simulink model "Encoder_B02"  (R2024b)
settings: Solver=FixedStepAuto  StartTime=0.0  StopTime=inf  FixedStep=0.01  RelTol=1e-3  EnableMultiTasking=on
libraries: stm32f4xxblockslib x10, stm32g4xxblockslib x9
settings Model: STM32="{\"EncoderBlockForG4\":[{\"ID\":\"Hi:51\"},{\"ID\":\"Hi:52\"},{\"ID\":\"Hi:61\"},{\"ID\":\"Hi:103\"},{\"ID\":\"Hi:104\"},{\"ID\":\"Hi:105\"},{\"ID\":\"Hi:147\"},{\"ID\":\"Hi:148\"},{\"ID\":\"Hi:149\"}],\"DigitalPortRead\":[{\"ID\":\"Hi:68\"},{\"ID\":\"Hi:69\"},{\"ID\":\"Hi:95\"},{\"ID\":\"Hi:96\"},{\"ID\":\"Hi:118\"},{\"ID\":\"Hi:119\"},{\"ID\":\"Hi:131\"},{\"ID\":\"Hi:132\"},{\"ID\":\"Hi:133\"},{\"ID\":\"Hi:134\"}]}"  SimulationMode=external  Creator=User  LastModifiedBy=User
settings OptimizationCC: DefaultParameterBehavior=Inlined  EnhancedBackFolding=on  PassReuseOutputArgsAs=Individual arguments  ZeroExternalMemoryAtStartup=off  ZeroInternalMemoryAtStartup=off  MaxStackSize=512  OptimizeBlockOrder=speed  DifferentSizesBufferReuse=on  OptimizationCustomize=off  EfficientTunableParamExpr=on
settings DebuggingCC: ParameterTunabilityLossMsg=error
settings HardwareCC: ProdBitPerPointer=32  ProdBitPerSizeT=32  ProdBitPerPtrDiffT=32  ProdLargestAtomicInteger=Long  ProdLargestAtomicFloat=Double  ProdWordSize=32  ProdLongLongMode=on  ProdHWDeviceType=ARM Compatible->ARM Cortex-M
settings SFSimCC: MATLABDynamicMemAlloc=off
settings RTWCC: Description=Embedded Coder  SystemTargetFile=ert.tlc  HardwareBoard=STM32G4xx Based  TemplateMakefile=ert_default_tmf  Toolchain=GNU Tools for ARM Embedded Processors
settings CodeAppCC: ForceParamTrailComments=on  IgnoreCustomStorageClasses=off  OperatorAnnotations=on  SimulinkDataObjDesc=on  SFDataObjDesc=on  InsertBlockDesc=on
settings ERTTargetCC: TargetLangStandard=C99 (ISO)  CodeReplacementLibrary=ARM Cortex-M  ExtModeTransport=3  ExtModeStaticAlloc=on  ExtModeStaticAllocSize=2048  ExtModeMexFile=ext_xcp  ExtModeIntrfLevel=Level2 - Open

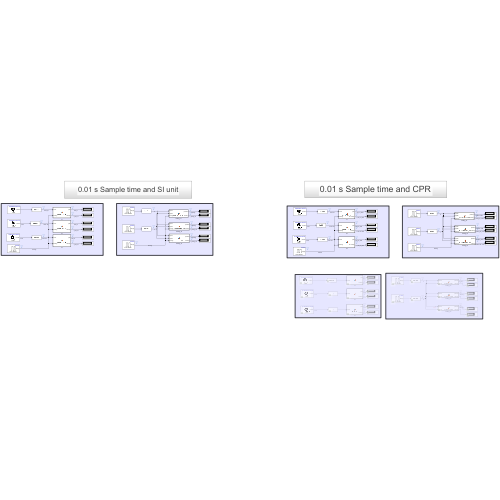
[thumbnail: Simulink's stored preview of the top-level diagram]
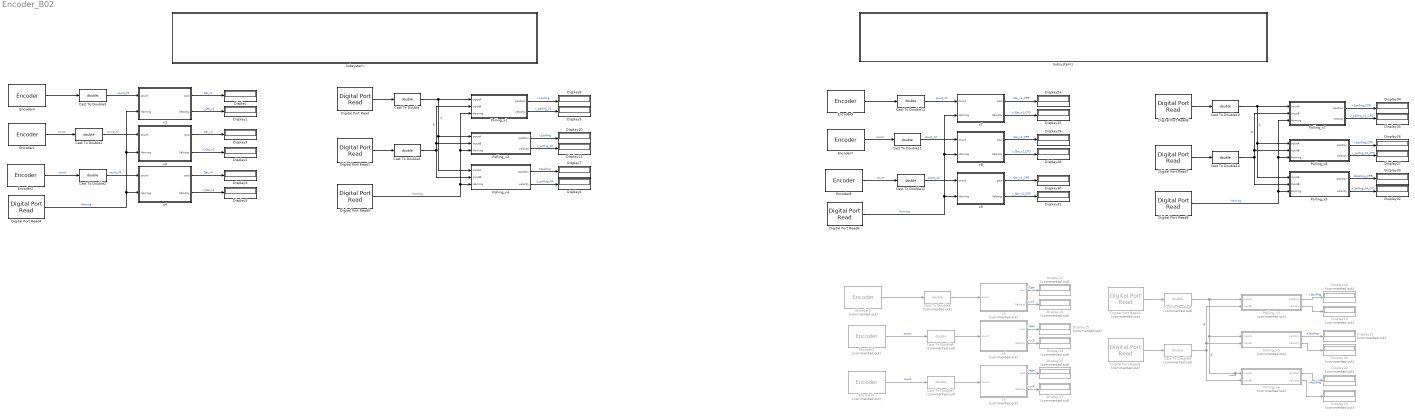
== system Encoder_B02 ==
  Cast To Double{,1..4,10..14} (10 alike) : DataTypeConversion  OutDataTypeStr=double  SaturateOnIntegerOverflow=off  RndMeth=Floor
  Cast To Double{5..9} (5 alike) : DataTypeConversion  Commented=on  OutDataTypeStr=double  SaturateOnIntegerOverflow=off  RndMeth=Floor
  Digital Port Read : stm32f4xxblockslib/Digital Port Read  PortName=GPIOB  PinNumber=[4]  ReadOperation=on  IOAsArray=on  SampleTime=-1  EnableSimPort=off  hoistedMaskSrc=ECSoC/ECSimCodegen/Digital Port Read
  Digital Port Read1 : stm32f4xxblockslib/Digital Port Read  PortName=GPIOB  PinNumber=[5]  ReadOperation=on  IOAsArray=on  SampleTime=-1  EnableSimPort=off  hoistedMaskSrc=ECSoC/ECSimCodegen/Digital Port Read
  Digital Port Read2 : stm32f4xxblockslib/Digital Port Read  Commented=on  PortName=GPIOB  PinNumber=[4]  ReadOperation=on  IOAsArray=on  SampleTime=-1  EnableSimPort=off  hoistedMaskSrc=ECSoC/ECSimCodegen/Digital Port Read
  Digital Port Read3 : stm32f4xxblockslib/Digital Port Read  Commented=on  PortName=GPIOB  PinNumber=[5]  ReadOperation=on  IOAsArray=on  SampleTime=-1  EnableSimPort=off  hoistedMaskSrc=ECSoC/ECSimCodegen/Digital Port Read
  Digital Port Read{4..5,8..9} (4 alike) : stm32f4xxblockslib/Digital Port Read  PortName=GPIOC  PinNumber=[13]  ReadOperation=on  IOAsArray=on  SampleTime=-1  EnableSimPort=off  hoistedMaskSrc=ECSoC/ECSimCodegen/Digital Port Read
  Digital Port Read6 : stm32f4xxblockslib/Digital Port Read  PortName=GPIOB  PinNumber=[4]  ReadOperation=on  IOAsArray=on  SampleTime=-1  EnableSimPort=off  hoistedMaskSrc=ECSoC/ECSimCodegen/Digital Port Read
  Digital Port Read7 : stm32f4xxblockslib/Digital Port Read  PortName=GPIOB  PinNumber=[5]  ReadOperation=on  IOAsArray=on  SampleTime=-1  EnableSimPort=off  hoistedMaskSrc=ECSoC/ECSimCodegen/Digital Port Read
  Display{,1..11,24..35} (24 alike) : Display
  Display{12..23} (12 alike) : Display  Commented=on
  Encoder1 : stm32g4xxblockslib/Encoder  TimerModule=TIM4  EnableResetInput=off  OutputCountAfterFirstIndex=off  OutputValidIndex=off  OutputDirection=off  OutputStatus=off  SampleTime=-1
  Encoder2 : stm32g4xxblockslib/Encoder  TimerModule=TIM8  EnableResetInput=off  OutputCountAfterFirstIndex=off  OutputValidIndex=off  OutputDirection=off  OutputStatus=off  SampleTime=-1
  Encoder3 : stm32g4xxblockslib/Encoder  Commented=on  TimerModule=TIM4  EnableResetInput=off  OutputCountAfterFirstIndex=off  OutputValidIndex=off  OutputDirection=off  OutputStatus=off  SampleTime=-1
  Encoder4 : stm32g4xxblockslib/Encoder  TimerModule=TIM3  EnableResetInput=off  OutputCountAfterFirstIndex=off  OutputValidIndex=off  OutputDirection=off  OutputStatus=off  SampleTime=-1
  Encoder5 : stm32g4xxblockslib/Encoder  Commented=on  TimerModule=TIM8  EnableResetInput=off  OutputCountAfterFirstIndex=off  OutputValidIndex=off  OutputDirection=off  OutputStatus=off  SampleTime=-1
  Encoder6 : stm32g4xxblockslib/Encoder  Commented=on  TimerModule=TIM3  EnableResetInput=off  OutputCountAfterFirstIndex=off  OutputValidIndex=off  OutputDirection=off  OutputStatus=off  SampleTime=-1
  Encoder7 : stm32g4xxblockslib/Encoder  TimerModule=TIM4  EnableResetInput=off  OutputCountAfterFirstIndex=off  OutputValidIndex=off  OutputDirection=off  OutputStatus=off  SampleTime=-1
  Encoder8 : stm32g4xxblockslib/Encoder  TimerModule=TIM8  EnableResetInput=off  OutputCountAfterFirstIndex=off  OutputValidIndex=off  OutputDirection=off  OutputStatus=off  SampleTime=-1
  Encoder9 : stm32g4xxblockslib/Encoder  TimerModule=TIM3  EnableResetInput=off  OutputCountAfterFirstIndex=off  OutputValidIndex=off  OutputDirection=off  OutputStatus=off  SampleTime=-1
  Polling_x1 : MATLAB Function  TreatAsAtomicUnit=on
  Polling_x2 : MATLAB Function  TreatAsAtomicUnit=on
  Polling_x3 : MATLAB Function  Commented=on  TreatAsAtomicUnit=on
  Polling_x4 : MATLAB Function  TreatAsAtomicUnit=on
  Polling_x5 : MATLAB Function  Commented=on  TreatAsAtomicUnit=on
  Polling_x6 : MATLAB Function  Commented=on  TreatAsAtomicUnit=on
  Polling_x7 : MATLAB Function  TreatAsAtomicUnit=on
  Polling_x8 : MATLAB Function  TreatAsAtomicUnit=on
  Polling_x9 : MATLAB Function  TreatAsAtomicUnit=on
  Subsystem : Subsystem
  Subsystem1 : Subsystem
  x1 : MATLAB Function  TreatAsAtomicUnit=on
  x2 : MATLAB Function  TreatAsAtomicUnit=on
  x3 : MATLAB Function  Commented=on  TreatAsAtomicUnit=on
  x4 : MATLAB Function  TreatAsAtomicUnit=on
  x5 : MATLAB Function  Commented=on  TreatAsAtomicUnit=on
  x6 : MATLAB Function  Commented=on  TreatAsAtomicUnit=on
  x7 : MATLAB Function  TreatAsAtomicUnit=on
  x8 : MATLAB Function  TreatAsAtomicUnit=on
  x9 : MATLAB Function  TreatAsAtomicUnit=on
  wires:
  Cast To Double2/1 -> x4/1(count)  "count_X4"
  Encoder2/1 -> Cast To Double2/1  "count"
  Encoder1/1 -> Cast To Double1/1  "count"
  Cast To Double1/1 -> x2/1(count)  "count_X2"
  Encoder4/1 -> Cast To Double3/1
  Cast To Double3/1 -> x1/1(count)  "count_X1"
  Digital Port Read/1 -> Cast To Double/1
  Digital Port Read1/1 -> Cast To Double4/1
  Cast To Double/1 -> Polling_x4/1(inputA), Polling_x2/1(inputA), Polling_x1/1(inputA)  "A"
  Cast To Double4/1 -> Polling_x4/2(inputB), Polling_x1/2(inputB), Polling_x2/2(inputB)  "B"
  x1/1(posi) -> Display/1  "Qei_x1"
  x1/2(Velocity) -> Display1/1  "v_Qei_x1"
  x2/1(posi) -> Display3/1  "Qei_x2"
  x2/2(Velocity) -> Display2/1  "v_Qei_x2"
  x4/1(posi) -> Display4/1  "Qei_x4"
  x4/2(Velocity) -> Display5/1  "v_Qei_x4"
  Polling_x4/2(velocity) -> Display6/1  "v_polling_X4"
  Polling_x4/1(position) -> Display7/1  "X4polling"
  Polling_x1/1(position) -> Display8/1  "x1polling"
  Polling_x1/2(velocity) -> Display9/1  "v_polling_X1"
  Polling_x2/1(position) -> Display10/1  "x2polling"
  Polling_x2/2(velocity) -> Display11/1  "v_polling_X2"
  Polling_x6/2(velocity) -> Display23/1
  Cast To Double9/1 -> Polling_x6/2(inputB), Polling_x3/2(inputB), Polling_x5/2(inputB)  "B"
  x6/2(Velocity) -> Display17/1  "v_x4"
  x6/1(posi) -> Display16/1  "x4qei"
  x5/1(posi) -> Display15/1  "x2qei"
  Polling_x5/1(position) -> Display21/1  "x2pulling"
  Polling_x6/1(position) -> Display22/1  "x4pulling"
  Encoder6/1 -> Cast To Double8/1
  Polling_x3/1(position) -> Display18/1  "x1pulling"
  Cast To Double7/1 -> x6/1(count)
  Cast To Double6/1 -> x5/1(count)
  Encoder5/1 -> Cast To Double7/1  "count"
  Digital Port Read3/1 -> Cast To Double9/1
  Encoder3/1 -> Cast To Double6/1  "count"
  x5/2(Velocity) -> Display14/1  "v_x2"
  x3/2(Velocity) -> Display13/1  "v_x1"
  Cast To Double8/1 -> x3/1(count)
  Polling_x3/2(velocity) -> Display19/1
  x3/1(posi) -> Display12/1  "x1qei"
  Cast To Double5/1 -> Polling_x6/1(inputA), Polling_x5/1(inputA), Polling_x3/1(inputA)  "A"
  Digital Port Read2/1 -> Cast To Double5/1
  Polling_x5/2(velocity) -> Display20/1
  Digital Port Read4/1 -> x1/2(Homing), x2/2(Homing), x4/2(Homing)  "Homing"
  Digital Port Read5/1 -> Polling_x1/3(Homing), Polling_x2/3(Homing), Polling_x4/3(Homing)  "Homing"
  Polling_x8/2(velocity) -> Display27/1  "v_polling_X2_CPS"
  Digital Port Read7/1 -> Cast To Double14/1
  x9/2(Velocity) -> Display31/1  "v_Qei_x4_CPS"
  x8/1(posi) -> Display29/1  "Qei_x2_CPR"
  Encoder8/1 -> Cast To Double12/1  "count"
  Cast To Double11/1 -> x8/1(count)  "count_X2"
  Polling_x9/1(position) -> Display33/1  "X4polling_CPR"
  Polling_x9/2(velocity) -> Display32/1  "v_polling_X4_CPS"
  Polling_x7/1(position) -> Display34/1  "x1polling_CPR"
  Encoder9/1 -> Cast To Double13/1
  Digital Port Read9/1 -> Polling_x7/3(Homing), Polling_x8/3(Homing), Polling_x9/3(Homing)  "Homing"
  Encoder7/1 -> Cast To Double11/1  "count"
  Cast To Double13/1 -> x7/1(count)  "count_X1"
  x7/2(Velocity) -> Display25/1  "v_Qei_x1_CPS"
  x8/2(Velocity) -> Display28/1  "v_Qei_x2_CPS"
  Cast To Double10/1 -> Polling_x9/1(inputA), Polling_x8/1(inputA), Polling_x7/1(inputA)  "A"
  Cast To Double12/1 -> x9/1(count)  "count_X4"
  x7/1(posi) -> Display24/1  "Qei_x1_CPR"
  Digital Port Read6/1 -> Cast To Double10/1
  Cast To Double14/1 -> Polling_x9/2(inputB), Polling_x7/2(inputB), Polling_x8/2(inputB)  "B"
  Polling_x7/2(velocity) -> Display35/1  "v_polling_X1_CPS"
  x9/1(posi) -> Display30/1  "Qei_x4_CPR"
  Digital Port Read8/1 -> x8/2(Homing), x7/2(Homing), x9/2(Homing)  "Homing"
  Polling_x8/1(position) -> Display26/1  "x2polling_CPR"

== system Encoder_B02/Subsystem ==
  note: 0.01 s Sample time and SI unit

== system Encoder_B02/Subsystem1 ==
  note: 0.01 s Sample time and CPR

== matlab function Encoder_B02/x5 ==
  data: count input; posi output; Velocity output
function [posi,Velocity] = encoder(count)

    persistent prev c;
    if isempty(prev)
        prev = 0;
        c = 0;
    end
    interval = 65520-mod(65520,24);
    delta_count = count - prev;
    if delta_count < (-interval/2)
        delta_count = delta_count + (interval); %Clockwise_Shift count+(66520-prev)
    elseif delta_count > (interval/2)
        delta_count = -interval + delta_count; %Couter_Clockwise_Shift -(66520-count)-prev
    end

    c = c + delta_count;
    prev = count;
    Velocity = delta_count*100;
    posi = c ;
end

== matlab function Encoder_B02/x6 ==
  data: count input; posi output; Velocity output
function [posi,Velocity] = encoder(count)

    persistent prev c;
    if isempty(prev)
        prev = 0;
        c = 0;
    end
    interval = 65520-mod(65520,24);
    delta_count = count - prev;
    if delta_count < (-interval/2)
        delta_count = delta_count + (interval); %Clockwise_Shift count+(66520-prev)
    elseif delta_count > (interval/2)
        delta_count = -interval + delta_count; %Couter_Clockwise_Shift -(66520-count)-prev
    end

    c = c + delta_count;
    prev = count;
    Velocity = delta_count*100;
    posi = c ;
end

== matlab function Encoder_B02/Polling_x7 ==
  data: inputA input; position output; inputB input; velocity output; Homing input
function [position,velocity]  = EncoderPolling_X1(inputA, inputB ,Homing)
    persistent prevA prevB count prev_count;
    
    % Initialize persistent 
    if isempty(prevA)
        prevA = inputA;
        prevB = inputB;
        count = 0;
        prev_count = 0;
    end

    % Detect changes 
    if (prevA == 0 && prevB == 0)
        if inputA == 1 && inputB == 0
            count = count + 1; % Clockwise 
        end
    elseif (prevA == 0 && prevB == 1)
        if inputA == 1 && inputB == 1
            count = count - 1; % Clockwise 
        end
    end

    % Update previous state
    prevA = inputA;
    prevB = inputB;

    % Output 
    position = count;
    velocity = (count-prev_count)*100;
    prev_count = count;
    if Homing == 1 
        position = 0;
        count = 0;
        prev_count = 0;
    end
end

== matlab function Encoder_B02/Polling_x8 ==
  data: inputA input; position output; inputB input; velocity output; Homing input
function [position,velocity] = EncoderPolling_X2(inputA, inputB ,Homing)
     persistent prevA prevB count prev_count;
    
    if isempty(prevA)
        prevA = inputA;
        prevB = inputB;
        count = 0;
        prev_count = 0;
    end

    if (prevA == 0 && prevB == 0)
        if inputA == 1 && inputB == 0
            count = count + 1; % Clockwise 
        end
    elseif (prevA == 0 && prevB == 1)
        if inputA == 1 && inputB == 1
            count = count - 1; % Clockwise 
        end
    elseif (prevA == 1 && prevB == 1)
        if inputA == 0 && inputB == 1
            count = count + 1; % Clockwise 
        end
    elseif (prevA == 1 && prevB == 0)
        if inputA == 0 && inputB == 0
            count = count - 1; % Clockwise 
        end
    end

    % Update Prev
    prevA = inputA;
    prevB = inputB;

    % Output
    position = count;
    velocity = (count-prev_count)*100;
    prev_count = count;
    if Homing == 1 
        position = 0;
        count = 0;
        prev_count = 0;
    end
end

== matlab function Encoder_B02/Polling_x9 ==
  data: inputA input; position output; inputB input; velocity output; Homing input
function [position,velocity] = EncoderPolling_X4(inputA, inputB ,Homing)
     persistent prevA prevB count prev_count;
    
    if isempty(prevA)
        prevA = inputA;
        prevB = inputB;
        count = 0;
        prev_count = 0;
    end
    if (prevA == 0 && prevB == 0)
        if inputA == 1 && inputB == 0
            count = count + 1; % Clockwise 
        end
        if inputA == 0 && inputB == 1
            count = count - 1; % Clockwise 
        end

    elseif (prevA == 0 && prevB == 1)
        if inputA == 1 && inputB == 1
            count = count - 1; % Clockwise 
        end
        if inputA == 0 && inputB == 0
            count = count + 1; % Clockwise 
        end

    elseif (prevA == 1 && prevB == 1)
        if inputA == 0 && inputB == 1
            count = count + 1; % Clockwise 
        end
        if inputA == 1 && inputB == 0
            count = count - 1; % Clockwise 
        end

    elseif (prevA == 1 && prevB == 0)
        if inputA == 0 && inputB == 0
            count = count - 1; % Clockwise 
        end
        if inputA == 1 && inputB == 1
            count = count + 1; % Clockwise 
        end
    end

    % Update Prev
    prevA = inputA;
    prevB = inputB;

    % Output
    position = count;
    velocity = (count-prev_count)*100;
    prev_count = count;
    if Homing == 1 
        position = 0;
        count = 0;
        prev_count = 0;
    end
end

== matlab function Encoder_B02/x2 ==
  data: count input; posi output; Velocity output; Homing input
function [posi,Velocity] = EncoderQEI_X2(count,Homing)

    persistent prev c;
    if isempty(prev)
        prev = 0;
        c = 0;
    end
    interval = 65520-mod(65520,48);
    delta_count = count - prev;
    if delta_count < (-interval/2)
        delta_count = delta_count + (interval); %Clockwise_Shift count+(66520-prev)
    elseif delta_count > (interval/2)
        delta_count = -interval + delta_count; %Couter_Clockwise_Shift -(66520-count)-prev
    end

    c = c + delta_count;
    prev = count;
    Velocity = delta_count*100*((2*pi)/48);
    posi = c*((2*pi)/48) ;
    if Homing == 1 
        prev = count;
        c = 0;
        posi = 0;
    end
end

== matlab function Encoder_B02/x7 ==
  data: count input; posi output; Velocity output; Homing input
function [posi,Velocity] = EncoderQEI_X1(count,Homing)

    persistent prev c;
    if isempty(prev)
        prev = 0;
        c = 0;
    end
    interval = 65520-mod(65520,24);
    delta_count = count - prev;
    if delta_count < (-interval/2)
        delta_count = delta_count + (interval); %Clockwise_Shift count+(66520-prev)
    elseif delta_count > (interval/2)
        delta_count = -interval + delta_count; %Couter_Clockwise_Shift -(66520-count)-prev
    end

    c = c + delta_count;
    prev = count;
    Velocity = delta_count*100;
    posi = c;
    if Homing == 1 
        prev = count;
        c = 0;
        posi = 0;
    end
end

== matlab function Encoder_B02/x8 ==
  data: count input; posi output; Velocity output; Homing input
function [posi,Velocity] = EncoderQEI_X2(count,Homing)

    persistent prev c;
    if isempty(prev)
        prev = 0;
        c = 0;
    end
    interval = 65520-mod(65520,24);
    delta_count = count - prev;
    if delta_count < (-interval/2)
        delta_count = delta_count + (interval); %Clockwise_Shift count+(66520-prev)
    elseif delta_count > (interval/2)
        delta_count = -interval + delta_count; %Couter_Clockwise_Shift -(66520-count)-prev
    end

    c = c + delta_count;
    prev = count;
    Velocity = delta_count*100;
    posi = c ;
    if Homing == 1 
        prev = count;
        c = 0;
        posi = 0;
    end
end

== matlab function Encoder_B02/x9 ==
  data: count input; posi output; Velocity output; Homing input
function [posi,Velocity] = EncoderQEI_X4(count,Homing)

    persistent prev c;
    if isempty(prev) 
        prev = 0;
        c = 0;
    end
    interval = 65520-mod(65520,24);
    delta_count = count - prev;
    if delta_count < (-interval/2)
        delta_count = delta_count + (interval); %Clockwise_Shift count+(66520-prev)
    elseif delta_count > (interval/2)
        delta_count = -interval + delta_count; %Couter_Clockwise_Shift -(66520-count)-prev
    end

    c = c + delta_count;
    prev = count;
    Velocity = delta_count*100;
    posi = c ;
    if Homing == 1 
        prev = count;
        c = 0;
        posi = 0;
    end
end

== matlab function Encoder_B02/Polling_x1 ==
  data: inputA input; position output; inputB input; velocity output; Homing input
function [position,velocity]  = EncoderPolling_X1(inputA, inputB ,Homing)
    persistent prevA prevB count prev_count;
    
    % Initialize persistent 
    if isempty(prevA)
        prevA = inputA;
        prevB = inputB;
        count = 0;
        prev_count = 0;
    end

    % Detect changes 
    if (prevA == 0 && prevB == 0)
        if inputA == 1 && inputB == 0
            count = count + 1; % Clockwise 
        end
    elseif (prevA == 0 && prevB == 1)
        if inputA == 1 && inputB == 1
            count = count - 1; % Clockwise 
        end
    end

    % Update previous state
    prevA = inputA;
    prevB = inputB;

    % Output 
    position = count*((2*pi)/2048);
    velocity = (count-prev_count)*100*((2*pi)/2048);
    prev_count = count;
    if Homing == 1 
        position = 0;
        count = 0;
        prev_count = 0;
    end
end

== matlab function Encoder_B02/x4 ==
  data: count input; posi output; Velocity output; Homing input
function [posi,Velocity] = EncoderQEI_X4(count,Homing)

    persistent prev c;
    if isempty(prev) 
        prev = 0;
        c = 0;
    end
    interval = 65520-mod(65520,96);
    delta_count = count - prev;
    if delta_count < (-interval/2)
        delta_count = delta_count + (interval); %Clockwise_Shift count+(66520-prev)
    elseif delta_count > (interval/2)
        delta_count = -interval + delta_count; %Couter_Clockwise_Shift -(66520-count)-prev
    end

    c = c + delta_count;
    prev = count;
    Velocity = delta_count*100*((2*pi)/96);
    posi = c*((2*pi)/96) ;
    if Homing == 1 
        prev = count;
        c = 0;
        posi = 0;
    end
end

== matlab function Encoder_B02/x1 ==
  data: count input; posi output; Velocity output; Homing input
function [posi,Velocity] = EncoderQEI_X1(count,Homing)

    persistent prev c;
    if isempty(prev)
        prev = 0;
        c = 0;
    end
    interval = 65520-mod(65520,24);
    delta_count = count - prev;
    if delta_count < (-interval/2)
        delta_count = delta_count + (interval);                                   %Clockwise_Shift count+(66520-prev)
    elseif delta_count > (interval/2)
        delta_count = -interval + delta_count;                                    %Couter_Clockwise_Shift -(66520-count)-prev
    end

    c = c + delta_count;
    prev = count;
    Velocity = delta_count*100*((2*pi)/24);
    posi = c*((2*pi)/24);
    if Homing == 1 
        prev = count;
        c = 0;
        posi = 0;
    end
end

== matlab function Encoder_B02/Polling_x2 ==
  data: inputA input; position output; inputB input; velocity output; Homing input
function [position,velocity] = EncoderPolling_X2(inputA, inputB ,Homing)
     persistent prevA prevB count prev_count;
    
    if isempty(prevA)
        prevA = inputA;
        prevB = inputB;
        count = 0;
        prev_count = 0;
    end

    if (prevA == 0 && prevB == 0)
        if inputA == 1 && inputB == 0
            count = count + 1; % Clockwise 
        end
    elseif (prevA == 0 && prevB == 1)
        if inputA == 1 && inputB == 1
            count = count - 1; % Clockwise 
        end
    elseif (prevA == 1 && prevB == 1)
        if inputA == 0 && inputB == 1
            count = count + 1; % Clockwise 
        end
    elseif (prevA == 1 && prevB == 0)
        if inputA == 0 && inputB == 0
            count = count - 1; % Clockwise 
        end
    end

    % Update Prev
    prevA = inputA;
    prevB = inputB;

    % Output
    position = count*((2*pi)/4048);
    velocity = (count-prev_count)*100*((2*pi)/4048);
    prev_count = count;
    if Homing == 1 
        position = 0;
        count = 0;
        prev_count = 0;
    end
end

== matlab function Encoder_B02/Polling_x4 ==
  data: inputA input; position output; inputB input; velocity output; Homing input
function [position,velocity] = EncoderPolling_X4(inputA, inputB ,Homing)
     persistent prevA prevB count prev_count;
    
    if isempty(prevA)
        prevA = inputA;
        prevB = inputB;
        count = 0;
        prev_count = 0;
    end
    if (prevA == 0 && prevB == 0)
        if inputA == 1 && inputB == 0
            count = count + 1; % Clockwise 
        end
        if inputA == 0 && inputB == 1
            count = count - 1; % Clockwise 
        end

    elseif (prevA == 0 && prevB == 1)
        if inputA == 1 && inputB == 1
            count = count - 1; % Clockwise 
        end
        if inputA == 0 && inputB == 0
            count = count + 1; % Clockwise 
        end

    elseif (prevA == 1 && prevB == 1)
        if inputA == 0 && inputB == 1
            count = count + 1; % Clockwise 
        end
        if inputA == 1 && inputB == 0
            count = count - 1; % Clockwise 
        end

    elseif (prevA == 1 && prevB == 0)
        if inputA == 0 && inputB == 0
            count = count - 1; % Clockwise 
        end
        if inputA == 1 && inputB == 1
            count = count + 1; % Clockwise 
        end
    end

    % Update Prev
    prevA = inputA;
    prevB = inputB;

    % Output
    position = count*((2*pi)/8192);
    velocity = (count-prev_count)*100*((2*pi)/8192);
    prev_count = count;
    if Homing == 1 
        position = 0;
        count = 0;
        prev_count = 0;
    end
end

== matlab function Encoder_B02/Polling_x3 ==
  data: inputA input; position output; inputB input; velocity output
function [position,velocity]  = readEncoderX1(inputA, inputB)
    persistent prevA prevB count prev_count;
    
    % Initialize persistent 
    if isempty(prevA)
        prevA = inputA;
        prevB = inputB;
        count = 0;
        prev_count = 0;
    end

    % Detect changes 
    if (prevA == 0 && prevB == 0)
        if inputA == 1 && inputB == 0
            count = count + 1; % Clockwise 
        end
    elseif (prevA == 0 && prevB == 1)
        if inputA == 1 && inputB == 1
            count = count - 1; % Clockwise 
        end
    end

    % Update previous state
    prevA = inputA;
    prevB = inputB;

    % Output 
    position = count;
    velocity = (count-prev_count)*100;
    prev_count = count;
end

== matlab function Encoder_B02/Polling_x5 ==
  data: inputA input; position output; inputB input; velocity output
function [position,velocity] = readEncoderX2(inputA, inputB)
     persistent prevA prevB count prev_count;
    
    if isempty(prevA)
        prevA = inputA;
        prevB = inputB;
        count = 0;
        prev_count = 0;
    end

    if (prevA == 0 && prevB == 0)
        if inputA == 1 && inputB == 0
            count = count + 1; % Clockwise 
        end
    elseif (prevA == 0 && prevB == 1)
        if inputA == 1 && inputB == 1
            count = count - 1; % Clockwise 
        end
    elseif (prevA == 1 && prevB == 1)
        if inputA == 0 && inputB == 1
            count = count + 1; % Clockwise 
        end
    elseif (prevA == 1 && prevB == 0)
        if inputA == 0 && inputB == 0
            count = count - 1; % Clockwise 
        end
    end

    % Update Prev
    prevA = inputA;
    prevB = inputB;

    % Output
    position = count;
    velocity = (count-prev_count)*100;
    prev_count = count;
end

== matlab function Encoder_B02/Polling_x6 ==
  data: inputA input; position output; inputB input; velocity output
function [position,velocity] = readEncoderX4(inputA, inputB)
     persistent prevA prevB count prev_count;
    
    if isempty(prevA)
        prevA = inputA;
        prevB = inputB;
        count = 0;
        prev_count = 0;
    end
    if (prevA == 0 && prevB == 0)
        if inputA == 1 && inputB == 0
            count = count + 1; % Clockwise 
        end
        if inputA == 0 && inputB == 1
            count = count - 1; % Clockwise 
        end

    elseif (prevA == 0 && prevB == 1)
        if inputA == 1 && inputB == 1
            count = count - 1; % Clockwise 
        end
        if inputA == 0 && inputB == 0
            count = count + 1; % Clockwise 
        end

    elseif (prevA == 1 && prevB == 1)
        if inputA == 0 && inputB == 1
            count = count + 1; % Clockwise 
        end
        if inputA == 1 && inputB == 0
            count = count - 1; % Clockwise 
        end

    elseif (prevA == 1 && prevB == 0)
        if inputA == 0 && inputB == 0
            count = count - 1; % Clockwise 
        end
        if inputA == 1 && inputB == 1
            count = count + 1; % Clockwise 
        end
    end

    % Update Prev
    prevA = inputA;
    prevB = inputB;

    % Output
    position = count;
    velocity = (count-prev_count)*100;
    prev_count = count;
end

== matlab function Encoder_B02/x3 ==
  data: count input; posi output; Velocity output
function [posi,Velocity] = encoder(count)

    persistent prev c;
    if isempty(prev)
        prev = 0;
        c = 0;
    end
    interval = 65520-mod(65520,24);
    delta_count = count - prev;
    if delta_count < (-interval/2)
        delta_count = delta_count + (interval); %Clockwise_Shift count+(66520-prev)
    elseif delta_count > (interval/2)
        delta_count = -interval + delta_count; %Couter_Clockwise_Shift -(66520-count)-prev
    end

    c = c + delta_count;
    prev = count;
    Velocity = delta_count*100;
    posi = c;
end
